simulink model "tbp_test"  (R2023b)
settings: Solver=ode113  StartTime=0.0  StopTime=period  RelTol=1e-13  AbsTol=1e-13
undefined symbols (not defined in the file): r0, v0
libraries: dyn_lib x1
settings Model: Creator=brent  LastModifiedBy=brent

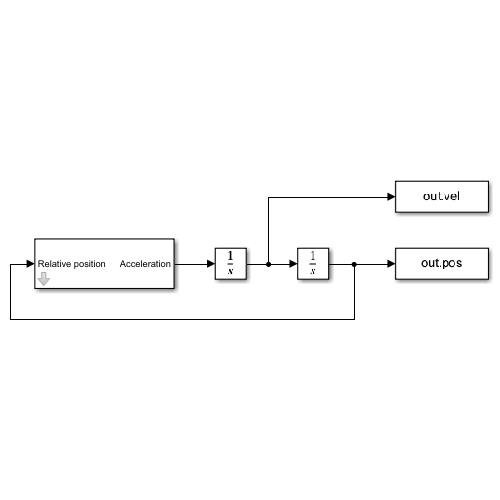
[thumbnail: Simulink's stored preview of the top-level diagram]
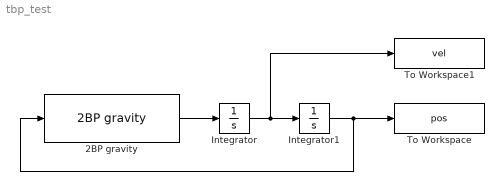
== system tbp_test ==
  2BP gravity : dyn_lib/2BP gravity  mu=mu
      settings: SourceProductName=Dynamics library
  Integrator : Integrator  InitialCondition=v0
  Integrator1 : Integrator  InitialCondition=r0
  To Workspace : ToWorkspace  VariableName=pos  SaveFormat=Timeseries  SampleTime=-1
  To Workspace1 : ToWorkspace  VariableName=vel  SaveFormat=Timeseries  SampleTime=-1
  wires:
  Integrator/1 -> To Workspace1/1, Integrator1/1
  Integrator1/1 -> To Workspace/1, 2BP gravity/1
  2BP gravity/1 -> Integrator/1
